simulink model "Xe_Model_Redo_June_26"  (R2018a)
settings: Solver=VariableStepAuto  StartTime=0.0  StopTime=5E5+96*60*60  RelTol=1e-3
values from neighbouring files (symbols this model uses):
  A_pipe = pi*r_pipe^2    (= 0.0126676869774)    [Startup_Script.m]
  alpha_FS = 0.517E-16    (= 5.17e-17)    [Startup_Script.m]
  alpha_G_R1 = 0.334E-17    (= 3.34e-18)    [Startup_Script.m]
  alpha_G_R2 = 0.699E-17    (= 6.99e-18)    [Startup_Script.m]
  alpha_G_R3 = 0.669E-17    (= 6.69e-18)    [Startup_Script.m]
  alpha_G_R4 = 0.791E-18    (= 7.91e-19)    [Startup_Script.m]
  D_g = 2.37E-9    (= 2.37e-09)    [Startup_Script.m]
  epsilon = 0.1    [Startup_Script.m]
  eta_b = 1E-4    (= 0.0001)    [Startup_Script.m]
  eta_fs = 1.2E-4    (= 0.00012)    [Startup_Script.m]
  f_cv = 0.004    [Startup_Script.m]
  FS_Mu_A = 4340    [Startup_Script.m]
  FS_Mu_K = 0.084    [Startup_Script.m]
  FS_Mu_MSRE = 0.007027    [Startup_Script.m]
  FS_rho_A = 3.628    [Startup_Script.m]
  FS_rho_B = 0.00066    [Startup_Script.m]
  FS_rho_MSRE = 2082    [Startup_Script.m]
  gamma_i = 0.0293524    [Startup_Script.m]
  gamma_te = 0.0322482    [Startup_Script.m]
  gamma_xe = 0.00257324    [Startup_Script.m]
  h_fc = 1.6    [Startup_Script.m]
  H_Xe_a = 5.713e-13    [Startup_Script.m]
  H_Xe_b = -7.937e-10    [Startup_Script.m]
  H_Xe_c = 2.809e-07    [Startup_Script.m]
  HX_r_Tube = ((0.5-0.042)/2)*2.54E-2    (= 0.0058166)    [Startup_Script.m]
  HX_XS = HX_N_Tubes*(pi*HX_r_Tube^2)    (= 0.0168999490356)    [Startup_Script.m]
  k_b = 1.3806E-23    (= 1.3806e-23)    [Startup_Script.m]
  lambda_i = 2.9306070546251702E-5    (= 2.93060705463e-05)    [Startup_Script.m]
  lambda_te = 0.036481430555786593    (= 0.0364814305558)    [Startup_Script.m]
  lambda_xe = 2.0924e-05    [Startup_Script.m]
  N_FC_R1 = 12    [Startup_Script.m]
  N_FC_R2 = 940    [Startup_Script.m]
  N_FC_R3 = 108    [Startup_Script.m]
  N_FC_R4 = 78    [Startup_Script.m]
  P_pump = 35420    [Startup_Script.m]
  phi0 = 3.98E+17    (= 3.98e+17)    [Startup_Script.m]
  phi_G_R_1 = mean(interp1(phi_G_R,phi_G_phi, linspace(0,r_g_r1)))    [Startup_Script.m]
  phi_G_R_2 = mean(interp1(phi_G_R,phi_G_phi, linspace(r_g_r1,r_g_r2)))    [Startup_Script.m]
  phi_G_R_3 = mean(interp1(phi_G_R,phi_G_phi, linspace(r_g_r2,r_g_r3)))    [Startup_Script.m]
  phi_G_R_4 = mean(interp1(phi_G_R,phi_G_phi, linspace(r_g_r3,r_g_r4)))    [Startup_Script.m]
  Q_strpr = 0.003155    [Startup_Script.m]
  Q_tot = 0.07571    [Startup_Script.m]
  r_b = 0.000254    [Startup_Script.m]
  r_fc = 0.79e-2    (= 0.0079)    [Startup_Script.m]
  r_pipe = (5E-2*2.54)/2    (= 0.0635)    [Startup_Script.m]
  r_xe = 2.16E-10    (= 2.16e-10)    [Startup_Script.m]
  Re_CA = 25800    [Startup_Script.m]
  Re_LH = 1E4    (= 10000)    [Startup_Script.m]
  Re_UH = 1E4    (= 10000)    [Startup_Script.m]
  sig_a_xe = 1.18E-22    (= 1.18e-22)    [Startup_Script.m]
  Sig_f = 0.15    [Startup_Script.m]
  T_CA_0 = T_INLET    (= 907.594444444)    [Startup_Script.m]
  T_FP_0 = T_OUTLET    (= 935.372222222)    [Startup_Script.m]
  T_FS_R_1_0 = mean(interp1(R_fs_m,T_fs_K, linspace(0,r_g_r1)))    [Startup_Script.m]
  T_FS_R_2_0 = mean(interp1(R_fs_m,T_fs_K, linspace(r_g_r1,r_g_r2)))    [Startup_Script.m]
  T_FS_R_3_0 = mean(interp1(R_fs_m,T_fs_K, linspace(r_g_r2,r_g_r3)))    [Startup_Script.m]
  T_FS_R_4_0 = mean(interp1(R_fs_m,T_fs_K, linspace(r_g_r3,r_g_r4)))    [Startup_Script.m]
  T_G_R_1_0 = mean(interp1(R_gr_m,T_gr_K, linspace(0,r_g_r1)))    [Startup_Script.m]
  T_HX_0 = 0.5*(T_OUTLET + T_INLET)    (= 921.483333333)    [Startup_Script.m]
  T_LH_0 = T_INLET    (= 907.594444444)    [Startup_Script.m]
  T_Mes = 928.15    [Startup_Script.m]
  T_P100_0 = T_OUTLET    (= 935.372222222)    [Startup_Script.m]
  T_P101_0 = T_OUTLET    (= 935.372222222)    [Startup_Script.m]
  T_P102_0 = T_INLET    (= 907.594444444)    [Startup_Script.m]
  T_Salt_0 = 900    [Startup_Script.m]
  T_UH_0 = T_OUTLET    (= 935.372222222)    [Startup_Script.m]
  U_FC_R1 = 0.607    [Startup_Script.m]
  U_FC_R2 = 0.183    [Startup_Script.m]
  U_FC_R3 = 0.454    [Startup_Script.m]
  U_FC_R4 = 0.250    (= 0.25)    [Startup_Script.m]
  V_CA_0 = 9.7*cubed_foot_to_cubed_meter    (= 0.274673445)    [Startup_Script.m]
  V_FP_0 = (0.9+3.2)*cubed_foot_to_cubed_meter    (= 0.116099085)    [Startup_Script.m]
  V_HX_0 = 6.1*cubed_foot_to_cubed_meter    (= 0.172732785)    [Startup_Script.m]
  V_LH_0 = 10.0*cubed_foot_to_cubed_meter    (= 0.2831685)    [Startup_Script.m]
  V_P100_0 = 2.1*cubed_foot_to_cubed_meter    (= 0.059465385)    [Startup_Script.m]
  V_P101_0 = 0.8*cubed_foot_to_cubed_meter    (= 0.02265348)    [Startup_Script.m]
  V_P102_0 = 2.2*cubed_foot_to_cubed_meter    (= 0.06229707)    [Startup_Script.m]
  V_R1_0 = V_Core_FS_0 *N_FC_R1/N_FC_tot    (= 0.00753107712766)    [Startup_Script.m]
  V_R2_0 = V_Core_FS_0 *N_FC_R2/N_FC_tot    (= 0.589934375)    [Startup_Script.m]
  V_R3_0 = V_Core_FS_0 *N_FC_R3/N_FC_tot    (= 0.0677796941489)    [Startup_Script.m]
  V_R4_0 = V_Core_FS_0 *N_FC_R4/N_FC_tot    (= 0.0489520013298)    [Startup_Script.m]
  V_UH_0 = 10.5*cubed_foot_to_cubed_meter    (= 0.297326925)    [Startup_Script.m]
undefined symbols (not defined in the file or in its folder): magnitude, V_CA, V_HX, V_P2, V_P3, V_R1, V_R2, V_R3, V_R4, V_UH
libraries: simulink x4, dspindex x4, dspstat3 x4, SignalEditorBlockLib x2
(part 2 of 11)

== system Xe_Model_Redo_June_26/Graphite /Graphite Region 3 ==
  N_Xe_FS : Inport
  Graphite MTC R1 : Subsystem
  Graphite Stringer : Subsystem
  Product : Product  Inputs=3
  C_Xe_GS_Max : Outport
  C_Xe_GS_Mean : Outport  Port=2
  Nd_Xe_FS->GS : Outport  Port=3
  wires:
  [U_FC_R3] -> Graphite MTC R1/2(U_FC [m/s])
  [phi_G_R_3] -> Graphite Stringer/2(phi)
  [T_G_R_3] -> Graphite MTC R1/1(T_Salt)
  Product/1 -> Nd_Xe_FS->GS/1
  [T_G_R_3] -> Graphite Stringer/1(T)
  N_Xe_FS/1 -> Graphite Stringer/4(N_XE_FS)
  Graphite Stringer/2(C_Xe_GS_Mean) -> C_Xe_GS_Mean/1
  Graphite Stringer/3(J_Xe_FS->GS) -> Product/1
  Graphite Stringer/1(C_Xe_GS_Max) -> C_Xe_GS_Max/1
  [A_1_FC] -> Product/2
  [N_FC_R3] -> Product/3
  Graphite MTC R1/1(k_m_g [m/s]) -> Graphite Stringer/3(k_m_g)

== system Xe_Model_Redo_June_26/Graphite /Graphite Region 4 ==
  N_Xe_FS : Inport
  Graphite MTC R1 : Subsystem
  Graphite Stringer : Subsystem
  Product : Product  Inputs=3
  C_Xe_GS_Max : Outport
  C_Xe_GS_Mean : Outport  Port=2
  Nd_Xe_FS->GS : Outport  Port=3
  wires:
  [U_FC_R4] -> Graphite MTC R1/2(U_FC [m/s])
  [phi_G_R_4] -> Graphite Stringer/2(phi)
  [T_G_R_4] -> Graphite MTC R1/1(T_Salt)
  Product/1 -> Nd_Xe_FS->GS/1
  [T_G_R_4] -> Graphite Stringer/1(T)
  N_Xe_FS/1 -> Graphite Stringer/4(N_XE_FS)
  Graphite Stringer/2(C_Xe_GS_Mean) -> C_Xe_GS_Mean/1
  Graphite Stringer/3(J_Xe_FS->GS) -> Product/1
  Graphite Stringer/1(C_Xe_GS_Max) -> C_Xe_GS_Max/1
  [A_1_FC] -> Product/2
  [N_FC_R4] -> Product/3
  Graphite MTC R1/1(k_m_g [m/s]) -> Graphite Stringer/3(k_m_g)

== system Xe_Model_Redo_June_26/I/I Decay ==
  N_I : Inport
  Product : Product
  Nd_I : Outport
  wires:
  Product/1 -> Nd_I/1
  [lambda_i] -> Product/2
  N_I/1 -> Product/1

== system Xe_Model_Redo_June_26/I/I From Fission ==
  Product : Product  Inputs=4
  Nd_I : Outport
  wires:
  [Sig_f] -> Product/4
  [phi0] -> Product/1
  [gamma_i] -> Product/2
  [V_IC] -> Product/3
  Product/1 -> Nd_I/1

== system Xe_Model_Redo_June_26/Te/Te Decay ==
  n_te : Inport
  Product : Product
  nd_te : Outport
  wires:
  Product/1 -> nd_te/1
  [lambda_te] -> Product/2
  n_te/1 -> Product/1

== system Xe_Model_Redo_June_26/Te/Te From Fission ==
  Product : Product  Inputs=4
  nd_te : Outport
  wires:
  [Sig_f] -> Product/4
  [phi0] -> Product/1
  [gamma_te] -> Product/2
  [V_IC] -> Product/3
  Product/1 -> nd_te/1

== system Xe_Model_Redo_June_26/Xe/Burnout ==
  note: Concentration in all of gas phase
  N_Xe : Inport
  Divide : Product  Inputs=*/
  Product1 : Product  Inputs=4
  Scope1 : Scope
  Scope2 : Scope
  Scope3 : Scope
  Nd_Xe : Outport
  wires:
  [V_FS_liq] -> Divide/2
  Divide/1 -> Product1/1
  [V_IC] -> Scope2/1, Product1/4
  Product1/1 -> Nd_Xe/1
  N_Xe/1 -> Divide/1
  [phi0] -> Scope3/1, Product1/2
  [sig_a_xe] -> Scope1/1, Product1/3

== system Xe_Model_Redo_June_26/Xe/Xe Decay ==
  N_Xe : Inport
  Product : Product
  Nd_Xe : Outport
  wires:
  Product/1 -> Nd_Xe/1
  [lambda_xe] -> Product/2
  N_Xe/1 -> Product/1

== system Xe_Model_Redo_June_26/Xe/Xe From Fission ==
  Product : Product  Inputs=4
  Scope1 : Scope
  Nd_Xe : Outport
  wires:
  [Sig_f] -> Product/4
  [phi0] -> Product/1
  [gamma_xe] -> Product/2
  [V_IC] -> Scope1/1, Product/3
  Product/1 -> Nd_Xe/1

== system Xe_Model_Redo_June_26/Xenon Stripper/Bubble Stripping ==
  Stripper Flowrate [m^3/sec] : Inport
  Bubble Density Bubbles /m^3 : Product  Inputs=*/
  Bubble Flow Rate [bubbles/sec] : Product
  Bubble Removal Rate [Bubbles /sec] : Product
  Bubble Volume Removal Rate [m^3 /sec] : Product
  C_B [atoms/m^3] : Subsystem
  xe removal rate via bubbles [atoms/sec] : Product
  Removal of xenon from bubbles : Outport
  wires:
  [V_CV_Tot] -> Bubble Density Bubbles /m^3/1
  [N_Xe_B] -> C_B [atoms/m^3]/1(N_Xe_B)
  [V_1_B] -> Bubble Density Bubbles /m^3/2
  Bubble Flow Rate [bubbles/sec]/1 -> Bubble Removal Rate [Bubbles /sec]/2
  [eta_b] -> Bubble Removal Rate [Bubbles /sec]/1
  Bubble Removal Rate [Bubbles /sec]/1 -> Bubble Volume Removal Rate [m^3 /sec]/2
  C_B [atoms/m^3]/1(C_Xe_B) -> xe removal rate via bubbles [atoms/sec]/2
  Bubble Density Bubbles /m^3/1 -> Bubble Flow Rate [bubbles/sec]/1
  Stripper Flowrate [m^3/sec]/1 -> Bubble Flow Rate [bubbles/sec]/2
  [V_1_B] -> Bubble Volume Removal Rate [m^3 /sec]/1
  Bubble Volume Removal Rate [m^3 /sec]/1 -> xe removal rate via bubbles [atoms/sec]/1
  xe removal rate via bubbles [atoms/sec]/1 -> Removal of xenon from bubbles/1

== system Xe_Model_Redo_June_26/Xenon Stripper/Fuel Salt Concentration atoms//m^3 ==
  N_FS : Inport
  divide : Product  Inputs=*/
  C_FS : Outport
  wires:
  divide/1 -> C_FS/1
  N_FS/1 -> divide/1
  [V_FS_liq] -> divide/2

== system Xe_Model_Redo_June_26/Xenon Stripper/Fuel Salt Stripping ==
  Stripper Fowrate [m^3/sec] : Inport
  Fuel Salt Concentration [atoms/m^3] : Inport  Port=2
  Product : Product
  atoms/sec : Product
  Fuel Salt Remvoal rate [atoms/sec] : Outport
  wires:
  Product/1 -> Fuel Salt Remvoal rate [atoms/sec]/1
  Fuel Salt Concentration [atoms/m^3]/1 -> atoms/sec/2
  Stripper Fowrate [m^3/sec]/1 -> atoms/sec/1
  atoms/sec/1 -> Product/2
  [eta_fs] -> Product/1

== system Xe_Model_Redo_June_26/Bubbles/Bubble Mass Transfer/Bubble Total KMA ==
  note: Cooling Annulus
  Display7 : Display
      settings: Format=short_e
  HX KMA : Subsystem
  KMA FP : Subsystem
  KMA_CA : Subsystem
  KMA_IC : Subsystem
  KMA_LH : Subsystem
  KMA_UH : Subsystem
  P1 KMA : Subsystem
  P2 KMA : Subsystem
  P3 KMA : Subsystem
  Sum1 : Sum  Inputs=+++++++++
  KMA : Outport
  wires:
  P2 KMA/1(kma) -> Sum1/7
  P1 KMA/1(kma) -> Sum1/5
  KMA_UH/1(kmA) -> Sum1/2
  KMA FP/1(KMA) -> Sum1/6
  KMA_LH/1(kmA) -> Sum1/4
  Sum1/1 -> Display7/1, KMA/1
  KMA_IC/1(kmA) -> Sum1/3
  HX KMA/1(KMA) -> Sum1/8
  KMA_CA/1(KMA) -> Sum1/1
  P3 KMA/1(kma) -> Sum1/9

== system Xe_Model_Redo_June_26/Bubbles/Bubble Mass Transfer/CA ==
  N_Xe FS : Inport
  N_Xe Gas Phase : Inport  Port=2
  T Node : Inport  Port=3
  V_Gas_Node : Inport  Port=4
  Fuel Salt Concentration1 : Subsystem
  "HRT*C_B " : Subsystem
  KMA_CA : Subsystem
  Multiply : Product
  Scope : Scope
  Scope1 : Scope
  Scope2 : Scope
  Subtract1 : Sum  Inputs=+-
  Nd_Xe : Outport
  wires:
  N_Xe FS/1 -> Fuel Salt Concentration1/1(N_FS)
  Multiply/1 -> Nd_Xe/1
  Subtract1/1 -> Scope2/1, Multiply/1
  Fuel Salt Concentration1/1(C_Xe Liq FS) -> Scope/1, Subtract1/1
  V_Gas_Node/1 -> KMA_CA/2(V Gas Node)
  "HRT*C_B "/1(HRT*(C_Xe in Gas Phase)) -> Scope1/1, Subtract1/2
  T Node/1 -> "HRT*C_B "/2(T Node), KMA_CA/1(T FS Node)
  N_Xe Gas Phase/1 -> "HRT*C_B "/1(N_Xe Gas Phase)
  KMA_CA/1(KMA) -> Multiply/2

== system Xe_Model_Redo_June_26/Bubbles/Bubble Mass Transfer/FP ==
  N_Xe FS : Inport
  N_Xe Gas Phase : Inport  Port=2
  T Node : Inport  Port=3
  V_Gas_Node : Inport  Port=4
  Fuel Salt Concentration1 : Subsystem
  "HRT*C_B " : Subsystem
  KMA_FP : Subsystem
  Multiply : Product
  Subtract1 : Sum  Inputs=+-
  Nd_Xe : Outport
  wires:
  N_Xe FS/1 -> Fuel Salt Concentration1/1(N_FS)
  Multiply/1 -> Nd_Xe/1
  Subtract1/1 -> Multiply/1
  Fuel Salt Concentration1/1(C_Xe Liq FS) -> Subtract1/1
  V_Gas_Node/1 -> KMA_FP/2(V Gas Node)
  "HRT*C_B "/1(HRT*(C_Xe in Gas Phase)) -> Subtract1/2
  T Node/1 -> "HRT*C_B "/2(T Node), KMA_FP/1(T FS Node)
  N_Xe Gas Phase/1 -> "HRT*C_B "/1(N_Xe Gas Phase)
  KMA_FP/1(KMA) -> Multiply/2

== system Xe_Model_Redo_June_26/Bubbles/Bubble Mass Transfer/G_R1 ==
  N_Xe FS : Inport
  N_Xe Gas Phase : Inport  Port=2
  T Node : Inport  Port=3
  V_Gas_Node : Inport  Port=4
  Fuel Salt Concentration1 : Subsystem
  "HRT*C_B " : Subsystem
  KMA_G_R1 : Subsystem
  Multiply : Product
  Subtract1 : Sum  Inputs=+-
  Nd_Xe : Outport
  wires:
  N_Xe FS/1 -> Fuel Salt Concentration1/1(N_FS)
  Multiply/1 -> Nd_Xe/1
  Subtract1/1 -> Multiply/1
  Fuel Salt Concentration1/1(C_Xe Liq FS) -> Subtract1/1
  V_Gas_Node/1 -> KMA_G_R1/2(V Gas Node)
  "HRT*C_B "/1(HRT*(C_Xe in Gas Phase)) -> Subtract1/2
  T Node/1 -> KMA_G_R1/1(T FS Node), "HRT*C_B "/2(T Node)
  N_Xe Gas Phase/1 -> "HRT*C_B "/1(N_Xe Gas Phase)
  KMA_G_R1/1(KMA) -> Multiply/2

== system Xe_Model_Redo_June_26/Bubbles/Bubble Mass Transfer/G_R2 ==
  N_Xe FS : Inport
  N_Xe Gas Phase : Inport  Port=2
  T Node : Inport  Port=3
  V_Gas_Node : Inport  Port=4
  Fuel Salt Concentration1 : Subsystem
  "HRT*C_B " : Subsystem
  KMA_G_R1 : Subsystem
  Multiply : Product
  Subtract1 : Sum  Inputs=+-
  Nd_Xe : Outport
  wires:
  N_Xe FS/1 -> Fuel Salt Concentration1/1(N_FS)
  Multiply/1 -> Nd_Xe/1
  Subtract1/1 -> Multiply/1
  Fuel Salt Concentration1/1(C_Xe Liq FS) -> Subtract1/1
  V_Gas_Node/1 -> KMA_G_R1/2(V Gas Node)
  "HRT*C_B "/1(HRT*(C_Xe in Gas Phase)) -> Subtract1/2
  T Node/1 -> KMA_G_R1/1(T FS Node), "HRT*C_B "/2(T Node)
  N_Xe Gas Phase/1 -> "HRT*C_B "/1(N_Xe Gas Phase)
  KMA_G_R1/1(KMA) -> Multiply/2

== system Xe_Model_Redo_June_26/Bubbles/Bubble Mass Transfer/G_R3 ==
  N_Xe FS : Inport
  N_Xe Gas Phase : Inport  Port=2
  T Node : Inport  Port=3
  V_Gas_Node : Inport  Port=4
  Fuel Salt Concentration1 : Subsystem
  "HRT*C_B " : Subsystem
  KMA_G_R1 : Subsystem
  Multiply : Product
  Subtract1 : Sum  Inputs=+-
  Nd_Xe : Outport
  wires:
  N_Xe FS/1 -> Fuel Salt Concentration1/1(N_FS)
  Multiply/1 -> Nd_Xe/1
  Subtract1/1 -> Multiply/1
  Fuel Salt Concentration1/1(C_Xe Liq FS) -> Subtract1/1
  V_Gas_Node/1 -> KMA_G_R1/2(V Gas Node)
  "HRT*C_B "/1(HRT*(C_Xe in Gas Phase)) -> Subtract1/2
  T Node/1 -> KMA_G_R1/1(T FS Node), "HRT*C_B "/2(T Node)
  N_Xe Gas Phase/1 -> "HRT*C_B "/1(N_Xe Gas Phase)
  KMA_G_R1/1(KMA) -> Multiply/2

== system Xe_Model_Redo_June_26/Bubbles/Bubble Mass Transfer/G_R4 ==
  N_Xe FS : Inport
  N_Xe Gas Phase : Inport  Port=2
  T Node : Inport  Port=3
  V_Gas_Node : Inport  Port=4
  Fuel Salt Concentration1 : Subsystem
  "HRT*C_B " : Subsystem
  KMA_G_R1 : Subsystem
  Multiply : Product
  Subtract1 : Sum  Inputs=+-
  Nd_Xe : Outport
  wires:
  N_Xe FS/1 -> Fuel Salt Concentration1/1(N_FS)
  Multiply/1 -> Nd_Xe/1
  Subtract1/1 -> Multiply/1
  Fuel Salt Concentration1/1(C_Xe Liq FS) -> Subtract1/1
  V_Gas_Node/1 -> KMA_G_R1/2(V Gas Node)
  "HRT*C_B "/1(HRT*(C_Xe in Gas Phase)) -> Subtract1/2
  T Node/1 -> KMA_G_R1/1(T FS Node), "HRT*C_B "/2(T Node)
  N_Xe Gas Phase/1 -> "HRT*C_B "/1(N_Xe Gas Phase)
  KMA_G_R1/1(KMA) -> Multiply/2

== system Xe_Model_Redo_June_26/Bubbles/Bubble Mass Transfer/HX ==
  N_Xe FS : Inport
  N_Xe Gas Phase : Inport  Port=2
  T Node : Inport  Port=3
  V_Gas_Node : Inport  Port=4
  Fuel Salt Concentration1 : Subsystem
  "HRT*C_B " : Subsystem
  KMA_HX : Subsystem
  Multiply : Product
  Subtract1 : Sum  Inputs=+-
  Nd_Xe : Outport
  wires:
  N_Xe FS/1 -> Fuel Salt Concentration1/1(N_FS)
  Multiply/1 -> Nd_Xe/1
  Subtract1/1 -> Multiply/1
  Fuel Salt Concentration1/1(C_Xe Liq FS) -> Subtract1/1
  V_Gas_Node/1 -> KMA_HX/2(V Gas Node)
  "HRT*C_B "/1(HRT*(C_Xe in Gas Phase)) -> Subtract1/2
  T Node/1 -> KMA_HX/1(T FS Node), "HRT*C_B "/2(T Node)
  N_Xe Gas Phase/1 -> "HRT*C_B "/1(N_Xe Gas Phase)
  KMA_HX/1(KMA) -> Multiply/2

== system Xe_Model_Redo_June_26/Bubbles/Bubble Mass Transfer/LH ==
  N_Xe FS : Inport
  N_Xe Gas Phase : Inport  Port=2
  T Node : Inport  Port=3
  V_Gas_Node : Inport  Port=4
  Fuel Salt Concentration1 : Subsystem
  "HRT*C_B " : Subsystem
  KMA_LH : Subsystem
  Multiply : Product
  Subtract1 : Sum  Inputs=+-
  Nd_Xe : Outport
  wires:
  N_Xe FS/1 -> Fuel Salt Concentration1/1(N_FS)
  Multiply/1 -> Nd_Xe/1
  Subtract1/1 -> Multiply/1
  Fuel Salt Concentration1/1(C_Xe Liq FS) -> Subtract1/1
  V_Gas_Node/1 -> KMA_LH/2(V Gas Node)
  "HRT*C_B "/1(HRT*(C_Xe in Gas Phase)) -> Subtract1/2
  T Node/1 -> "HRT*C_B "/2(T Node), KMA_LH/1(T FS Node)
  N_Xe Gas Phase/1 -> "HRT*C_B "/1(N_Xe Gas Phase)
  KMA_LH/1(KMA) -> Multiply/2

== system Xe_Model_Redo_June_26/Bubbles/Bubble Mass Transfer/P100 ==
  N_Xe FS : Inport
  N_Xe Gas Phase : Inport  Port=2
  T Node : Inport  Port=3
  V_Gas_Node : Inport  Port=4
  Fuel Salt Concentration1 : Subsystem
  "HRT*C_B " : Subsystem
  KMA_P100 : Subsystem
  Multiply : Product
  Subtract1 : Sum  Inputs=+-
  Nd_Xe : Outport
  wires:
  N_Xe FS/1 -> Fuel Salt Concentration1/1(N_FS)
  Multiply/1 -> Nd_Xe/1
  Subtract1/1 -> Multiply/1
  Fuel Salt Concentration1/1(C_Xe Liq FS) -> Subtract1/1
  V_Gas_Node/1 -> KMA_P100/2(V Gas Node)
  "HRT*C_B "/1(HRT*(C_Xe in Gas Phase)) -> Subtract1/2
  T Node/1 -> KMA_P100/1(T FS Node), "HRT*C_B "/2(T Node)
  N_Xe Gas Phase/1 -> "HRT*C_B "/1(N_Xe Gas Phase)
  KMA_P100/1(KMA) -> Multiply/2

== system Xe_Model_Redo_June_26/Bubbles/Bubble Mass Transfer/P101 ==
  N_Xe FS : Inport
  N_Xe Gas Phase : Inport  Port=2
  T Node : Inport  Port=3
  V_Gas_Node : Inport  Port=4
  Fuel Salt Concentration1 : Subsystem
  "HRT*C_B " : Subsystem
  KMA_P101 : Subsystem
  Multiply : Product
  Subtract1 : Sum  Inputs=+-
  Nd_Xe : Outport
  wires:
  N_Xe FS/1 -> Fuel Salt Concentration1/1(N_FS)
  Multiply/1 -> Nd_Xe/1
  Subtract1/1 -> Multiply/1
  Fuel Salt Concentration1/1(C_Xe Liq FS) -> Subtract1/1
  V_Gas_Node/1 -> KMA_P101/2(V Gas Node)
  "HRT*C_B "/1(HRT*(C_Xe in Gas Phase)) -> Subtract1/2
  T Node/1 -> KMA_P101/1(T FS Node), "HRT*C_B "/2(T Node)
  N_Xe Gas Phase/1 -> "HRT*C_B "/1(N_Xe Gas Phase)
  KMA_P101/1(KMA) -> Multiply/2

== system Xe_Model_Redo_June_26/Bubbles/Bubble Mass Transfer/P102 ==
  N_Xe FS : Inport
  N_Xe Gas Phase : Inport  Port=2
  T Node : Inport  Port=3
  V_Gas_Node : Inport  Port=4
  Fuel Salt Concentration1 : Subsystem
  "HRT*C_B " : Subsystem
  KMA_P102 : Subsystem
  Multiply : Product
  Subtract1 : Sum  Inputs=+-
  Nd_Xe : Outport
  wires:
  N_Xe FS/1 -> Fuel Salt Concentration1/1(N_FS)
  Multiply/1 -> Nd_Xe/1
  Subtract1/1 -> Multiply/1
  Fuel Salt Concentration1/1(C_Xe Liq FS) -> Subtract1/1
  V_Gas_Node/1 -> KMA_P102/2(V Gas Node)
  "HRT*C_B "/1(HRT*(C_Xe in Gas Phase)) -> Subtract1/2
  T Node/1 -> KMA_P102/1(T FS Node), "HRT*C_B "/2(T Node)
  N_Xe Gas Phase/1 -> "HRT*C_B "/1(N_Xe Gas Phase)
  KMA_P102/1(KMA) -> Multiply/2

== system Xe_Model_Redo_June_26/Bubbles/Bubble Mass Transfer/UH ==
  N_Xe FS : Inport
  N_Xe Gas Phase : Inport  Port=2
  T Node : Inport  Port=3
  V_Gas_Node : Inport  Port=4
  Fuel Salt Concentration1 : Subsystem
  "HRT*C_B " : Subsystem
  KMA_UH : Subsystem
  Multiply : Product
  Subtract1 : Sum  Inputs=+-
  Nd_Xe : Outport
  wires:
  N_Xe FS/1 -> Fuel Salt Concentration1/1(N_FS)
  Multiply/1 -> Nd_Xe/1
  Subtract1/1 -> Multiply/1
  Fuel Salt Concentration1/1(C_Xe Liq FS) -> Subtract1/1
  V_Gas_Node/1 -> KMA_UH/2(V Gas Node)
  "HRT*C_B "/1(HRT*(C_Xe in Gas Phase)) -> Subtract1/2
  T Node/1 -> "HRT*C_B "/2(T Node), KMA_UH/1(T FS Node)
  N_Xe Gas Phase/1 -> "HRT*C_B "/1(N_Xe Gas Phase)
  KMA_UH/1(KMA) -> Multiply/2

== system Xe_Model_Redo_June_26/CONSTANTS/V CA/Current Density ==
  T_Salt [k] : Inport
  Cantor F1 Density : Subsystem
  Cantor F1 Density1 : Subsystem
  Constant3 : Constant  Value=T_Mes
  Constant4 : Constant  Value=FS_rho_MSRE
  Divide1 : Product  Inputs=*/
  Product1 : Product
  rho_FS [kg/m^3] : Outport
  wires:
  Divide1/1 -> Product1/2
  Cantor F1 Density1/1(rho [kg/m^3]) -> Divide1/2
  Constant4/1 -> Product1/1
  Cantor F1 Density/1(rho [kg/m^3]) -> Divide1/1
  Product1/1 -> rho_FS [kg/m^3]/1
  Constant3/1 -> Cantor F1 Density1/1(T_Salt [k])
  T_Salt [k]/1 -> Cantor F1 Density/1(T_Salt [k])

== system Xe_Model_Redo_June_26/CONSTANTS/V CA/Gain Gain ==
  Vol. Gas 0 : Inport
  T : Inport  Port=2
  "T_0 " : Inport  Port=3
  Divide : Product  Inputs=*/
  Multiply : Product
  V Gas : Outport
  wires:
  "T_0 "/1 -> Divide/2
  T/1 -> Divide/1
  Multiply/1 -> V Gas/1
  Divide/1 -> Multiply/2
  Vol. Gas 0/1 -> Multiply/1

== system Xe_Model_Redo_June_26/CONSTANTS/V CA/Reference Density ==
  T_Salt [k] : Inport
  Cantor F1 Density : Subsystem
  Cantor F1 Density1 : Subsystem
  Constant3 : Constant  Value=T_Mes
  Constant4 : Constant  Value=FS_rho_MSRE
  Divide1 : Product  Inputs=*/
  Product1 : Product
  rho_FS [kg/m^3] : Outport
  wires:
  Divide1/1 -> Product1/2
  Cantor F1 Density1/1(rho [kg/m^3]) -> Divide1/2
  Constant4/1 -> Product1/1
  Cantor F1 Density/1(rho [kg/m^3]) -> Divide1/1
  Product1/1 -> rho_FS [kg/m^3]/1
  Constant3/1 -> Cantor F1 Density1/1(T_Salt [k])
  T_Salt [k]/1 -> Cantor F1 Density/1(T_Salt [k])

== system Xe_Model_Redo_June_26/CONSTANTS/V FP/Current Density ==
  T_Salt [k] : Inport
  Cantor F1 Density : Subsystem
  Cantor F1 Density1 : Subsystem
  Constant3 : Constant  Value=T_Mes
  Constant4 : Constant  Value=FS_rho_MSRE
  Divide1 : Product  Inputs=*/
  Product1 : Product
  rho_FS [kg/m^3] : Outport
  wires:
  Divide1/1 -> Product1/2
  Cantor F1 Density1/1(rho [kg/m^3]) -> Divide1/2
  Constant4/1 -> Product1/1
  Cantor F1 Density/1(rho [kg/m^3]) -> Divide1/1
  Product1/1 -> rho_FS [kg/m^3]/1
  Constant3/1 -> Cantor F1 Density1/1(T_Salt [k])
  T_Salt [k]/1 -> Cantor F1 Density/1(T_Salt [k])

== system Xe_Model_Redo_June_26/CONSTANTS/V FP/Gain Gain ==
  Vol. Gas 0 : Inport
  T : Inport  Port=2
  "T_0 " : Inport  Port=3
  Divide : Product  Inputs=*/
  Multiply : Product
  V Gas : Outport
  wires:
  "T_0 "/1 -> Divide/2
  T/1 -> Divide/1
  Multiply/1 -> V Gas/1
  Divide/1 -> Multiply/2
  Vol. Gas 0/1 -> Multiply/1

== system Xe_Model_Redo_June_26/CONSTANTS/V FP/Reference Density ==
  T_Salt [k] : Inport
  Cantor F1 Density : Subsystem
  Cantor F1 Density1 : Subsystem
  Constant3 : Constant  Value=T_Mes
  Constant4 : Constant  Value=FS_rho_MSRE
  Divide1 : Product  Inputs=*/
  Product1 : Product
  rho_FS [kg/m^3] : Outport
  wires:
  Divide1/1 -> Product1/2
  Cantor F1 Density1/1(rho [kg/m^3]) -> Divide1/2
  Constant4/1 -> Product1/1
  Cantor F1 Density/1(rho [kg/m^3]) -> Divide1/1
  Product1/1 -> rho_FS [kg/m^3]/1
  Constant3/1 -> Cantor F1 Density1/1(T_Salt [k])
  T_Salt [k]/1 -> Cantor F1 Density/1(T_Salt [k])

== system Xe_Model_Redo_June_26/CONSTANTS/V FP1/Current Density ==
  T_Salt [k] : Inport
  Cantor F1 Density : Subsystem
  Cantor F1 Density1 : Subsystem
  Constant3 : Constant  Value=T_Mes
  Constant4 : Constant  Value=FS_rho_MSRE
  Divide1 : Product  Inputs=*/
  Product1 : Product
  rho_FS [kg/m^3] : Outport
  wires:
  Divide1/1 -> Product1/2
  Cantor F1 Density1/1(rho [kg/m^3]) -> Divide1/2
  Constant4/1 -> Product1/1
  Cantor F1 Density/1(rho [kg/m^3]) -> Divide1/1
  Product1/1 -> rho_FS [kg/m^3]/1
  Constant3/1 -> Cantor F1 Density1/1(T_Salt [k])
  T_Salt [k]/1 -> Cantor F1 Density/1(T_Salt [k])

== system Xe_Model_Redo_June_26/CONSTANTS/V FP1/Gain Gain ==
  Vol. Gas 0 : Inport
  T : Inport  Port=2
  "T_0 " : Inport  Port=3
  Divide : Product  Inputs=*/
  Multiply : Product
  V Gas : Outport
  wires:
  "T_0 "/1 -> Divide/2
  T/1 -> Divide/1
  Multiply/1 -> V Gas/1
  Divide/1 -> Multiply/2
  Vol. Gas 0/1 -> Multiply/1

== system Xe_Model_Redo_June_26/CONSTANTS/V FP1/Reference Density ==
  T_Salt [k] : Inport
  Cantor F1 Density : Subsystem
  Cantor F1 Density1 : Subsystem
  Constant3 : Constant  Value=T_Mes
  Constant4 : Constant  Value=FS_rho_MSRE
  Divide1 : Product  Inputs=*/
  Product1 : Product
  rho_FS [kg/m^3] : Outport
  wires:
  Divide1/1 -> Product1/2
  Cantor F1 Density1/1(rho [kg/m^3]) -> Divide1/2
  Constant4/1 -> Product1/1
  Cantor F1 Density/1(rho [kg/m^3]) -> Divide1/1
  Product1/1 -> rho_FS [kg/m^3]/1
  Constant3/1 -> Cantor F1 Density1/1(T_Salt [k])
  T_Salt [k]/1 -> Cantor F1 Density/1(T_Salt [k])

== system Xe_Model_Redo_June_26/CONSTANTS/V HX/Current Density ==
  T_Salt [k] : Inport
  Cantor F1 Density : Subsystem
  Cantor F1 Density1 : Subsystem
  Constant3 : Constant  Value=T_Mes
  Constant4 : Constant  Value=FS_rho_MSRE
  Divide1 : Product  Inputs=*/
  Product1 : Product
  rho_FS [kg/m^3] : Outport
  wires:
  Divide1/1 -> Product1/2
  Cantor F1 Density1/1(rho [kg/m^3]) -> Divide1/2
  Constant4/1 -> Product1/1
  Cantor F1 Density/1(rho [kg/m^3]) -> Divide1/1
  Product1/1 -> rho_FS [kg/m^3]/1
  Constant3/1 -> Cantor F1 Density1/1(T_Salt [k])
  T_Salt [k]/1 -> Cantor F1 Density/1(T_Salt [k])

== system Xe_Model_Redo_June_26/CONSTANTS/V HX/Gain Gain ==
  Vol. Gas 0 : Inport
  T : Inport  Port=2
  "T_0 " : Inport  Port=3
  Divide : Product  Inputs=*/
  Multiply : Product
  V Gas : Outport
  wires:
  "T_0 "/1 -> Divide/2
  T/1 -> Divide/1
  Multiply/1 -> V Gas/1
  Divide/1 -> Multiply/2
  Vol. Gas 0/1 -> Multiply/1

== system Xe_Model_Redo_June_26/CONSTANTS/V HX/Reference Density ==
  T_Salt [k] : Inport
  Cantor F1 Density : Subsystem
  Cantor F1 Density1 : Subsystem
  Constant3 : Constant  Value=T_Mes
  Constant4 : Constant  Value=FS_rho_MSRE
  Divide1 : Product  Inputs=*/
  Product1 : Product
  rho_FS [kg/m^3] : Outport
  wires:
  Divide1/1 -> Product1/2
  Cantor F1 Density1/1(rho [kg/m^3]) -> Divide1/2
  Constant4/1 -> Product1/1
  Cantor F1 Density/1(rho [kg/m^3]) -> Divide1/1
  Product1/1 -> rho_FS [kg/m^3]/1
  Constant3/1 -> Cantor F1 Density1/1(T_Salt [k])
  T_Salt [k]/1 -> Cantor F1 Density/1(T_Salt [k])

== system Xe_Model_Redo_June_26/CONSTANTS/V LH/Current Density ==
  T_Salt [k] : Inport
  Cantor F1 Density : Subsystem
  Cantor F1 Density1 : Subsystem
  Constant3 : Constant  Value=T_Mes
  Constant4 : Constant  Value=FS_rho_MSRE
  Divide1 : Product  Inputs=*/
  Product1 : Product
  rho_FS [kg/m^3] : Outport
  wires:
  Divide1/1 -> Product1/2
  Cantor F1 Density1/1(rho [kg/m^3]) -> Divide1/2
  Constant4/1 -> Product1/1
  Cantor F1 Density/1(rho [kg/m^3]) -> Divide1/1
  Product1/1 -> rho_FS [kg/m^3]/1
  Constant3/1 -> Cantor F1 Density1/1(T_Salt [k])
  T_Salt [k]/1 -> Cantor F1 Density/1(T_Salt [k])

== system Xe_Model_Redo_June_26/CONSTANTS/V LH/Gain Gain ==
  Vol. Gas 0 : Inport
  T : Inport  Port=2
  "T_0 " : Inport  Port=3
  Divide : Product  Inputs=*/
  Multiply : Product
  V Gas : Outport
  wires:
  "T_0 "/1 -> Divide/2
  T/1 -> Divide/1
  Multiply/1 -> V Gas/1
  Divide/1 -> Multiply/2
  Vol. Gas 0/1 -> Multiply/1

== system Xe_Model_Redo_June_26/CONSTANTS/V LH/Reference Density ==
  T_Salt [k] : Inport
  Cantor F1 Density : Subsystem
  Cantor F1 Density1 : Subsystem
  Constant3 : Constant  Value=T_Mes
  Constant4 : Constant  Value=FS_rho_MSRE
  Divide1 : Product  Inputs=*/
  Product1 : Product
  rho_FS [kg/m^3] : Outport
  wires:
  Divide1/1 -> Product1/2
  Cantor F1 Density1/1(rho [kg/m^3]) -> Divide1/2
  Constant4/1 -> Product1/1
  Cantor F1 Density/1(rho [kg/m^3]) -> Divide1/1
  Product1/1 -> rho_FS [kg/m^3]/1
  Constant3/1 -> Cantor F1 Density1/1(T_Salt [k])
  T_Salt [k]/1 -> Cantor F1 Density/1(T_Salt [k])

== system Xe_Model_Redo_June_26/CONSTANTS/V P100/Current Density ==
  T_Salt [k] : Inport
  Cantor F1 Density : Subsystem
  Cantor F1 Density1 : Subsystem
  Constant3 : Constant  Value=T_Mes
  Constant4 : Constant  Value=FS_rho_MSRE
  Divide1 : Product  Inputs=*/
  Product1 : Product
  rho_FS [kg/m^3] : Outport
  wires:
  Divide1/1 -> Product1/2
  Cantor F1 Density1/1(rho [kg/m^3]) -> Divide1/2
  Constant4/1 -> Product1/1
  Cantor F1 Density/1(rho [kg/m^3]) -> Divide1/1
  Product1/1 -> rho_FS [kg/m^3]/1
  Constant3/1 -> Cantor F1 Density1/1(T_Salt [k])
  T_Salt [k]/1 -> Cantor F1 Density/1(T_Salt [k])

== system Xe_Model_Redo_June_26/CONSTANTS/V P100/Gain Gain ==
  Vol. Gas 0 : Inport
  T : Inport  Port=2
  "T_0 " : Inport  Port=3
  Divide : Product  Inputs=*/
  Multiply : Product
  V Gas : Outport
  wires:
  "T_0 "/1 -> Divide/2
  T/1 -> Divide/1
  Multiply/1 -> V Gas/1
  Divide/1 -> Multiply/2
  Vol. Gas 0/1 -> Multiply/1

== system Xe_Model_Redo_June_26/CONSTANTS/V P100/Reference Density ==
  T_Salt [k] : Inport
  Cantor F1 Density : Subsystem
  Cantor F1 Density1 : Subsystem
  Constant3 : Constant  Value=T_Mes
  Constant4 : Constant  Value=FS_rho_MSRE
  Divide1 : Product  Inputs=*/
  Product1 : Product
  rho_FS [kg/m^3] : Outport
  wires:
  Divide1/1 -> Product1/2
  Cantor F1 Density1/1(rho [kg/m^3]) -> Divide1/2
  Constant4/1 -> Product1/1
  Cantor F1 Density/1(rho [kg/m^3]) -> Divide1/1
  Product1/1 -> rho_FS [kg/m^3]/1
  Constant3/1 -> Cantor F1 Density1/1(T_Salt [k])
  T_Salt [k]/1 -> Cantor F1 Density/1(T_Salt [k])

== system Xe_Model_Redo_June_26/CONSTANTS/V P101/Current Density ==
  T_Salt [k] : Inport
  Cantor F1 Density : Subsystem
  Cantor F1 Density1 : Subsystem
  Constant3 : Constant  Value=T_Mes
  Constant4 : Constant  Value=FS_rho_MSRE
  Divide1 : Product  Inputs=*/
  Product1 : Product
  rho_FS [kg/m^3] : Outport
  wires:
  Divide1/1 -> Product1/2
  Cantor F1 Density1/1(rho [kg/m^3]) -> Divide1/2
  Constant4/1 -> Product1/1
  Cantor F1 Density/1(rho [kg/m^3]) -> Divide1/1
  Product1/1 -> rho_FS [kg/m^3]/1
  Constant3/1 -> Cantor F1 Density1/1(T_Salt [k])
  T_Salt [k]/1 -> Cantor F1 Density/1(T_Salt [k])

== system Xe_Model_Redo_June_26/CONSTANTS/V P101/Gain Gain ==
  Vol. Gas 0 : Inport
  T : Inport  Port=2
  "T_0 " : Inport  Port=3
  Divide : Product  Inputs=*/
  Multiply : Product
  V Gas : Outport
  wires:
  "T_0 "/1 -> Divide/2
  T/1 -> Divide/1
  Multiply/1 -> V Gas/1
  Divide/1 -> Multiply/2
  Vol. Gas 0/1 -> Multiply/1

== system Xe_Model_Redo_June_26/CONSTANTS/V P101/Reference Density ==
  T_Salt [k] : Inport
  Cantor F1 Density : Subsystem
  Cantor F1 Density1 : Subsystem
  Constant3 : Constant  Value=T_Mes
  Constant4 : Constant  Value=FS_rho_MSRE
  Divide1 : Product  Inputs=*/
  Product1 : Product
  rho_FS [kg/m^3] : Outport
  wires:
  Divide1/1 -> Product1/2
  Cantor F1 Density1/1(rho [kg/m^3]) -> Divide1/2
  Constant4/1 -> Product1/1
  Cantor F1 Density/1(rho [kg/m^3]) -> Divide1/1
  Product1/1 -> rho_FS [kg/m^3]/1
  Constant3/1 -> Cantor F1 Density1/1(T_Salt [k])
  T_Salt [k]/1 -> Cantor F1 Density/1(T_Salt [k])

== system Xe_Model_Redo_June_26/CONSTANTS/V P102/Current Density ==
  T_Salt [k] : Inport
  Cantor F1 Density : Subsystem
  Cantor F1 Density1 : Subsystem
  Constant3 : Constant  Value=T_Mes
  Constant4 : Constant  Value=FS_rho_MSRE
  Divide1 : Product  Inputs=*/
  Product1 : Product
  rho_FS [kg/m^3] : Outport
  wires:
  Divide1/1 -> Product1/2
  Cantor F1 Density1/1(rho [kg/m^3]) -> Divide1/2
  Constant4/1 -> Product1/1
  Cantor F1 Density/1(rho [kg/m^3]) -> Divide1/1
  Product1/1 -> rho_FS [kg/m^3]/1
  Constant3/1 -> Cantor F1 Density1/1(T_Salt [k])
  T_Salt [k]/1 -> Cantor F1 Density/1(T_Salt [k])

== system Xe_Model_Redo_June_26/CONSTANTS/V P102/Gain Gain ==
  Vol. Gas 0 : Inport
  T : Inport  Port=2
  "T_0 " : Inport  Port=3
  Divide : Product  Inputs=*/
  Multiply : Product
  V Gas : Outport
  wires:
  "T_0 "/1 -> Divide/2
  T/1 -> Divide/1
  Multiply/1 -> V Gas/1
  Divide/1 -> Multiply/2
  Vol. Gas 0/1 -> Multiply/1

== system Xe_Model_Redo_June_26/CONSTANTS/V P102/Reference Density ==
  T_Salt [k] : Inport
  Cantor F1 Density : Subsystem
  Cantor F1 Density1 : Subsystem
  Constant3 : Constant  Value=T_Mes
  Constant4 : Constant  Value=FS_rho_MSRE
  Divide1 : Product  Inputs=*/
  Product1 : Product
  rho_FS [kg/m^3] : Outport
  wires:
  Divide1/1 -> Product1/2
  Cantor F1 Density1/1(rho [kg/m^3]) -> Divide1/2
  Constant4/1 -> Product1/1
  Cantor F1 Density/1(rho [kg/m^3]) -> Divide1/1
  Product1/1 -> rho_FS [kg/m^3]/1
  Constant3/1 -> Cantor F1 Density1/1(T_Salt [k])
  T_Salt [k]/1 -> Cantor F1 Density/1(T_Salt [k])

== system Xe_Model_Redo_June_26/CONSTANTS/V R1/Current Density ==
  T_Salt [k] : Inport
  Cantor F1 Density : Subsystem
  Cantor F1 Density1 : Subsystem
  Constant3 : Constant  Value=T_Mes
  Constant4 : Constant  Value=FS_rho_MSRE
  Divide1 : Product  Inputs=*/
  Product1 : Product
  rho_FS [kg/m^3] : Outport
  wires:
  Divide1/1 -> Product1/2
  Cantor F1 Density1/1(rho [kg/m^3]) -> Divide1/2
  Constant4/1 -> Product1/1
  Cantor F1 Density/1(rho [kg/m^3]) -> Divide1/1
  Product1/1 -> rho_FS [kg/m^3]/1
  Constant3/1 -> Cantor F1 Density1/1(T_Salt [k])
  T_Salt [k]/1 -> Cantor F1 Density/1(T_Salt [k])

== system Xe_Model_Redo_June_26/CONSTANTS/V R1/Gain Gain ==
  Vol. Gas 0 : Inport
  T : Inport  Port=2
  "T_0 " : Inport  Port=3
  Divide : Product  Inputs=*/
  Multiply : Product
  V Gas : Outport
  wires:
  "T_0 "/1 -> Divide/2
  T/1 -> Divide/1
  Multiply/1 -> V Gas/1
  Divide/1 -> Multiply/2
  Vol. Gas 0/1 -> Multiply/1

== system Xe_Model_Redo_June_26/CONSTANTS/V R1/Reference Density ==
  T_Salt [k] : Inport
  Cantor F1 Density : Subsystem
  Cantor F1 Density1 : Subsystem
  Constant3 : Constant  Value=T_Mes
  Constant4 : Constant  Value=FS_rho_MSRE
  Divide1 : Product  Inputs=*/
  Product1 : Product
  rho_FS [kg/m^3] : Outport
  wires:
  Divide1/1 -> Product1/2
  Cantor F1 Density1/1(rho [kg/m^3]) -> Divide1/2
  Constant4/1 -> Product1/1
  Cantor F1 Density/1(rho [kg/m^3]) -> Divide1/1
  Product1/1 -> rho_FS [kg/m^3]/1
  Constant3/1 -> Cantor F1 Density1/1(T_Salt [k])
  T_Salt [k]/1 -> Cantor F1 Density/1(T_Salt [k])

== system Xe_Model_Redo_June_26/CONSTANTS/V R2/Current Density ==
  T_Salt [k] : Inport
  Cantor F1 Density : Subsystem
  Cantor F1 Density1 : Subsystem
  Constant3 : Constant  Value=T_Mes
  Constant4 : Constant  Value=FS_rho_MSRE
  Divide1 : Product  Inputs=*/
  Product1 : Product
  rho_FS [kg/m^3] : Outport
  wires:
  Divide1/1 -> Product1/2
  Cantor F1 Density1/1(rho [kg/m^3]) -> Divide1/2
  Constant4/1 -> Product1/1
  Cantor F1 Density/1(rho [kg/m^3]) -> Divide1/1
  Product1/1 -> rho_FS [kg/m^3]/1
  Constant3/1 -> Cantor F1 Density1/1(T_Salt [k])
  T_Salt [k]/1 -> Cantor F1 Density/1(T_Salt [k])

== system Xe_Model_Redo_June_26/CONSTANTS/V R2/Gain Gain ==
  Vol. Gas 0 : Inport
  T : Inport  Port=2
  "T_0 " : Inport  Port=3
  Divide : Product  Inputs=*/
  Multiply : Product
  V Gas : Outport
  wires:
  "T_0 "/1 -> Divide/2
  T/1 -> Divide/1
  Multiply/1 -> V Gas/1
  Divide/1 -> Multiply/2
  Vol. Gas 0/1 -> Multiply/1

== system Xe_Model_Redo_June_26/CONSTANTS/V R2/Reference Density ==
  T_Salt [k] : Inport
  Cantor F1 Density : Subsystem
  Cantor F1 Density1 : Subsystem
  Constant3 : Constant  Value=T_Mes
  Constant4 : Constant  Value=FS_rho_MSRE
  Divide1 : Product  Inputs=*/
  Product1 : Product
  rho_FS [kg/m^3] : Outport
  wires:
  Divide1/1 -> Product1/2
  Cantor F1 Density1/1(rho [kg/m^3]) -> Divide1/2
  Constant4/1 -> Product1/1
  Cantor F1 Density/1(rho [kg/m^3]) -> Divide1/1
  Product1/1 -> rho_FS [kg/m^3]/1
  Constant3/1 -> Cantor F1 Density1/1(T_Salt [k])
  T_Salt [k]/1 -> Cantor F1 Density/1(T_Salt [k])

== system Xe_Model_Redo_June_26/CONSTANTS/V R3/Current Density ==
  T_Salt [k] : Inport
  Cantor F1 Density : Subsystem
  Cantor F1 Density1 : Subsystem
  Constant3 : Constant  Value=T_Mes
  Constant4 : Constant  Value=FS_rho_MSRE
  Divide1 : Product  Inputs=*/
  Product1 : Product
  rho_FS [kg/m^3] : Outport
  wires:
  Divide1/1 -> Product1/2
  Cantor F1 Density1/1(rho [kg/m^3]) -> Divide1/2
  Constant4/1 -> Product1/1
  Cantor F1 Density/1(rho [kg/m^3]) -> Divide1/1
  Product1/1 -> rho_FS [kg/m^3]/1
  Constant3/1 -> Cantor F1 Density1/1(T_Salt [k])
  T_Salt [k]/1 -> Cantor F1 Density/1(T_Salt [k])

== system Xe_Model_Redo_June_26/CONSTANTS/V R3/Gain Gain ==
  Vol. Gas 0 : Inport
  T : Inport  Port=2
  "T_0 " : Inport  Port=3
  Divide : Product  Inputs=*/
  Multiply : Product
  V Gas : Outport
  wires:
  "T_0 "/1 -> Divide/2
  T/1 -> Divide/1
  Multiply/1 -> V Gas/1
  Divide/1 -> Multiply/2
  Vol. Gas 0/1 -> Multiply/1

== system Xe_Model_Redo_June_26/CONSTANTS/V R3/Reference Density ==
  T_Salt [k] : Inport
  Cantor F1 Density : Subsystem
  Cantor F1 Density1 : Subsystem
  Constant3 : Constant  Value=T_Mes
  Constant4 : Constant  Value=FS_rho_MSRE
  Divide1 : Product  Inputs=*/
  Product1 : Product
  rho_FS [kg/m^3] : Outport
  wires:
  Divide1/1 -> Product1/2
  Cantor F1 Density1/1(rho [kg/m^3]) -> Divide1/2
  Constant4/1 -> Product1/1
  Cantor F1 Density/1(rho [kg/m^3]) -> Divide1/1
  Product1/1 -> rho_FS [kg/m^3]/1
  Constant3/1 -> Cantor F1 Density1/1(T_Salt [k])
  T_Salt [k]/1 -> Cantor F1 Density/1(T_Salt [k])

== system Xe_Model_Redo_June_26/CONSTANTS/V R4/Current Density ==
  T_Salt [k] : Inport
  Cantor F1 Density : Subsystem
  Cantor F1 Density1 : Subsystem
  Constant3 : Constant  Value=T_Mes
  Constant4 : Constant  Value=FS_rho_MSRE
  Divide1 : Product  Inputs=*/
  Product1 : Product
  rho_FS [kg/m^3] : Outport
  wires:
  Divide1/1 -> Product1/2
  Cantor F1 Density1/1(rho [kg/m^3]) -> Divide1/2
  Constant4/1 -> Product1/1
  Cantor F1 Density/1(rho [kg/m^3]) -> Divide1/1
  Product1/1 -> rho_FS [kg/m^3]/1
  Constant3/1 -> Cantor F1 Density1/1(T_Salt [k])
  T_Salt [k]/1 -> Cantor F1 Density/1(T_Salt [k])

== system Xe_Model_Redo_June_26/CONSTANTS/V R4/Gain Gain ==
  Vol. Gas 0 : Inport
  T : Inport  Port=2
  "T_0 " : Inport  Port=3
  Divide : Product  Inputs=*/
  Multiply : Product
  V Gas : Outport
  wires:
  "T_0 "/1 -> Divide/2
  T/1 -> Divide/1
  Multiply/1 -> V Gas/1
  Divide/1 -> Multiply/2
  Vol. Gas 0/1 -> Multiply/1

== system Xe_Model_Redo_June_26/CONSTANTS/V R4/Reference Density ==
  T_Salt [k] : Inport
  Cantor F1 Density : Subsystem
  Cantor F1 Density1 : Subsystem
  Constant3 : Constant  Value=T_Mes
  Constant4 : Constant  Value=FS_rho_MSRE
  Divide1 : Product  Inputs=*/
  Product1 : Product
  rho_FS [kg/m^3] : Outport
  wires:
  Divide1/1 -> Product1/2
  Cantor F1 Density1/1(rho [kg/m^3]) -> Divide1/2
  Constant4/1 -> Product1/1
  Cantor F1 Density/1(rho [kg/m^3]) -> Divide1/1
  Product1/1 -> rho_FS [kg/m^3]/1
  Constant3/1 -> Cantor F1 Density1/1(T_Salt [k])
  T_Salt [k]/1 -> Cantor F1 Density/1(T_Salt [k])

== system Xe_Model_Redo_June_26/CONSTANTS/V UH/Current Density ==
  T_Salt [k] : Inport
  Cantor F1 Density : Subsystem
  Cantor F1 Density1 : Subsystem
  Constant3 : Constant  Value=T_Mes
  Constant4 : Constant  Value=FS_rho_MSRE
  Divide1 : Product  Inputs=*/
  Product1 : Product
  rho_FS [kg/m^3] : Outport
  wires:
  Divide1/1 -> Product1/2
  Cantor F1 Density1/1(rho [kg/m^3]) -> Divide1/2
  Constant4/1 -> Product1/1
  Cantor F1 Density/1(rho [kg/m^3]) -> Divide1/1
  Product1/1 -> rho_FS [kg/m^3]/1
  Constant3/1 -> Cantor F1 Density1/1(T_Salt [k])
  T_Salt [k]/1 -> Cantor F1 Density/1(T_Salt [k])

== system Xe_Model_Redo_June_26/CONSTANTS/V UH/Gain Gain ==
  Vol. Gas 0 : Inport
  T : Inport  Port=2
  "T_0 " : Inport  Port=3
  Divide : Product  Inputs=*/
  Multiply : Product
  V Gas : Outport
  wires:
  "T_0 "/1 -> Divide/2
  T/1 -> Divide/1
  Multiply/1 -> V Gas/1
  Divide/1 -> Multiply/2
  Vol. Gas 0/1 -> Multiply/1

== system Xe_Model_Redo_June_26/CONSTANTS/V UH/Reference Density ==
  T_Salt [k] : Inport
  Cantor F1 Density : Subsystem
  Cantor F1 Density1 : Subsystem
  Constant3 : Constant  Value=T_Mes
  Constant4 : Constant  Value=FS_rho_MSRE
  Divide1 : Product  Inputs=*/
  Product1 : Product
  rho_FS [kg/m^3] : Outport
  wires:
  Divide1/1 -> Product1/2
  Cantor F1 Density1/1(rho [kg/m^3]) -> Divide1/2
  Constant4/1 -> Product1/1
  Cantor F1 Density/1(rho [kg/m^3]) -> Divide1/1
  Product1/1 -> rho_FS [kg/m^3]/1
  Constant3/1 -> Cantor F1 Density1/1(T_Salt [k])
  T_Salt [k]/1 -> Cantor F1 Density/1(T_Salt [k])

== system Xe_Model_Redo_June_26/Graphite /Graphite Region 1/Graphite MTC R1 ==
  note: Diemnsionless Numbers
  note: Thermophysical Properties
  T_Salt : Inport
  U_FC [m/s] : Inport  Port=2
  Constant : Constant  Value=0.023
  Constant1 : Constant  Value=0.8
  Constant2 : Constant  Value=0.4
  Density W Scaling : Subsystem
  Display : Display
  Divide : Product  Inputs=*/
  Gain : Gain  Gain=2
  Mass Diffusion Coeffecient [m^2 /s] : Subsystem
  Math Function : Math  Operator=pow  SaturateOnIntegerOverflow=on
  Math Function1 : Math  Operator=pow  SaturateOnIntegerOverflow=on
  Product : Product
  Reynolds Number : Subsystem
  Schmidt Number : Subsystem
  Sherwood Number : Product  Inputs=3
  Viscosity W Scaling : Subsystem
  k_m_g [m/s] : Outport
  wires:
  [D_FS_Local] -> Divide/1
  Constant2/1 -> Math Function1/2
  [r_fc] -> Gain/1
  Constant/1 -> Sherwood Number/1
  Sherwood Number/1 -> Product/1
  [Sc_FC_Local] -> Math Function1/1
  Divide/1 -> Product/2
  Math Function/1 -> Sherwood Number/2
  Constant1/1 -> Math Function/2
  Product/1 -> k_m_g [m/s]/1
  [Re_FC_Local] -> Math Function/1
  Math Function1/1 -> Sherwood Number/3
  Viscosity W Scaling/1(mu [Pa-s]) -> Mass Diffusion Coeffecient [m^2 /s]/1(Mu), [Mu_FS_Local]
  Density W Scaling/1(rho_FS [kg/m^3]) -> [Rho_FS_Local]
  Mass Diffusion Coeffecient [m^2 /s]/1(D [m^2/s]) -> [D_FS_Local]
  T_Salt/1 -> Mass Diffusion Coeffecient [m^2 /s]/2(T_Salt [k]), Density W Scaling/1(T_Salt [k]), Viscosity W Scaling/1(T_Salt [k])
  Schmidt Number/1(Sc) -> [Sc_FC_Local]
  Reynolds Number/1(Re) -> Display/1, [Re_FC_Local]
  U_FC [m/s]/1 -> Reynolds Number/1(Flow_Velocity [m/s])
  [Rho_FS_Local] -> Reynolds Number/2(rho [kg/m^3])
  [Mu_FS_Local] -> Reynolds Number/3(mu [Pa s])
  [Mu_FS_Local] -> Schmidt Number/1(mu [Pa s])
  [Rho_FS_Local] -> Schmidt Number/2(rho [kg/m^3])
  [D_FS_Local] -> Schmidt Number/3(D [m^2/s])
  Gain/1 -> Divide/2

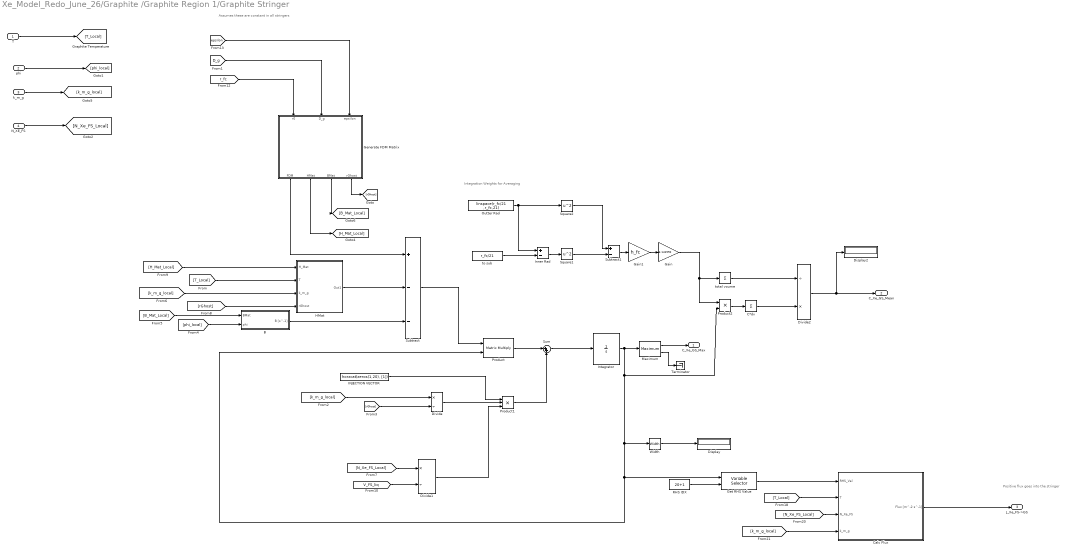
== system Xe_Model_Redo_June_26/Graphite /Graphite Region 1/Graphite Stringer ==
  note: Integration Weights for Averaging
  note: Assumes these are constant in all stringers
  note: Positive flux goes into the stringer
  T : Inport
  phi : Inport  Port=2
  k_m_g : Inport  Port=3
  N_XE_FS : Inport  Port=4
  B : Subsystem
  C*dv : Sum  Inputs=+
  Calc Flux : Subsystem
  Display : Display
  Display2 : Display
  Divide : Product  Inputs=*/
  Divide1 : Product  Inputs=*/
  Divide2 : Product  Inputs=/*
  Gain : Gain  Gain=3.141592
  Gain1 : Gain  Gain=h_fc
  "Generate FDM Matrix " : MATLAB Function  TreatAsAtomicUnit=on
  Get RHS Value : dspindex/Variable Selector  NumInputs=1  rowsOrCols=Rows  IdxMode=Variable  Elements=[1 3]  ZerOneIdxMode=One-based  errmode=Clip Index  FillMode=on  FillValues=0
  HMat : Subsystem
  INJECTION VECTOR : Constant  Value=horzcat(zeros(1,20), [1])
  Inner Rad : Sum  Inputs=+-
  Integrator : Integrator
  Maximum : dspstat3/Maximum  operation=maximum  fcn=Value and Index  indexBase=One  operateOver=Each column  Dimension=1  InputProcessing=Columns as channels (frame based)  reset=None  roiEnable=off  roiType=Rectangles  roiPortion=Entire ROI  roiOutput=Individual statistics for each ROI  roiFlag=off  roundingMode=Floor  overflowMode=off  accumDataTypeStr=Inherit: Same as product output  accumLastDataTypeStr=Inherit: Same as product output
  Outter Rad : Constant  Value=linspace(r_fc/21 ,r_fc,21)
  Product : Product  Multiplication=Matrix(*)
  Product1 : Product  Inputs=3
  Product2 : Product
  RHS IDX : Constant  Value=20+1
  Square1 : Math  Operator=square  SaturateOnIntegerOverflow=on
  Square2 : Math  Operator=square  SaturateOnIntegerOverflow=on
  Subtract : Sum  Inputs=+--
  Subtract1 : Sum  Inputs=+-
  Sum : Sum  Inputs=|++
  Terminator : Terminator
  Width : Width
  to sub : Constant  Value=r_fc/21
  total voume : Sum  Inputs=+
  C_Xe_GS_Max : Outport
  C_Xe_GS_Mean : Outport  Port=2
  J_Xe_FS->GS : Outport  Port=3
  wires:
  Get RHS Value/1 -> Calc Flux/1(RHS_Val)
  Calc Flux/1("Flux [m^-2 s^-1] ") -> J_Xe_FS->GS/1
  HMat/1(Out1) -> Subtract/2
  Maximum/1 -> C_Xe_GS_Max/1
  [rGhost] -> Divide/2
  Divide/1 -> Product1/2
  "Generate FDM Matrix "/1(FDM) -> Subtract/1
  "Generate FDM Matrix "/4(rGhost) -> [rGhost]
  [B_Mat_Local] -> B/1(BMat)
  phi/1 -> [phi_local]
  Subtract/1 -> Product/1
  Divide1/1 -> Product1/3
  Integrator/1 -> Product2/2, Width/1, Product/2, Get RHS Value/1, Maximum/1
  INJECTION VECTOR/1 -> Product1/1
  Product/1 -> Sum/1
  [T_Local] -> HMat/2(T)
  [epsilon] -> "Generate FDM Matrix "/3(epsilon)
  k_m_g/1 -> [k_m_g_local]
  [phi_local] -> B/2(phi)
  [k_m_g_local] -> HMat/3(k_m_g)
  [D_g] -> "Generate FDM Matrix "/2(D_g)
  "Generate FDM Matrix "/3(BMat) -> [B_Mat_Local]
  T/1 -> [T_Local]
  "Generate FDM Matrix "/2(HMat) -> [H_Mat_Local]
  [H_Mat_Local] -> HMat/1(H_Mat)
  [rGhost] -> HMat/4(rGhost)
  [k_m_g_local] -> Divide/1
  [r_fc] -> "Generate FDM Matrix "/1(r0)
  B/1("B [s^-1] ") -> Subtract/3
  Product1/1 -> Sum/2
  Sum/1 -> Integrator/1
  [V_FS_liq] -> Divide1/2
  RHS IDX/1 -> Get RHS Value/2
  [T_Local] -> Calc Flux/2(T)
  N_XE_FS/1 -> [N_Xe_FS_Local]
  [N_Xe_FS_Local] -> Divide1/1
  [k_m_g_local] -> Calc Flux/4(k_m_g)
  [N_Xe_FS_Local] -> Calc Flux/3(N_Xe_FS)
  Width/1 -> Display/1
  Outter Rad/1 -> Inner Rad/1, Square2/1
  Subtract1/1 -> Gain1/1
  Square1/1 -> Subtract1/2
  Square2/1 -> Subtract1/1
  Gain1/1 -> Gain/1
  to sub/1 -> Inner Rad/2
  Inner Rad/1 -> Square1/1
  Gain/1 -> Product2/1, total voume/1
  total voume/1 -> Divide2/1
  Product2/1 -> C*dv/1
  Divide2/1 -> Display2/1, C_Xe_GS_Mean/1
  C*dv/1 -> Divide2/2
  Maximum/2 -> Terminator/1

== system Xe_Model_Redo_June_26/Graphite /Graphite Region 1/Lumped Parameter Graphite Model ==
  PDE : Inport
  In2 : Inport  Port=2
  In3 : Inport  Port=3
  In4 : Inport  Port=4
  Burnout : Subsystem
  Constant : Constant  Value=h_fc
  Constant1 : Constant  Value=3.141592
  Divide : Product  Inputs=*/
  Integrator : Integrator
  Mux : Mux  Inputs=2
  Product1 : Product  Inputs=3
  Square1 : Math  Operator=square  SaturateOnIntegerOverflow=on
  Subsystem : Subsystem
  Sum : Sum  Inputs=+--
  To Workspace : ToWorkspace  VariableName=toSave_PDE  SampleTime=-1
  To Workspace1 : ToWorkspace  VariableName=toSave_LP  SampleTime=-1
  Xe Decay : Subsystem
  Out1 : Outport
  tag scope: V_GS=global
  wires:
  In3/1 -> Subsystem/2(MTC)
  [V_GS] -> Divide/2
  Constant/1 -> Product1/2
  [A_1_FC] -> Subsystem/5(A)
  Divide/1 -> To Workspace1/1, Mux/2  "LP"
  Product1/1 -> [V_GS]
  In2/1 -> Subsystem/1(T)
  Square1/1 -> Product1/1
  PDE/1 -> To Workspace/1, Mux/1
  [r_fc] -> Square1/1
  Subsystem/1(Out1) -> Sum/1
  Burnout/1(Nd_Xe) -> Sum/2
  Integrator/1 -> Divide/1, Xe Decay/1(N_Xe_B), Subsystem/4(N_Xe_G), Burnout/1(N_Xe_G)
  Xe Decay/1(Nd_Xe) -> Sum/3
  [phi_G_R_1] -> Burnout/2(Phi)
  Sum/1 -> Integrator/1
  Constant1/1 -> Product1/3
  In4/1 -> Subsystem/3(V_FS_liq)
  Mux/1 -> Out1/1

== system Xe_Model_Redo_June_26/Graphite /Graphite Region 2/Graphite MTC R1 ==
  note: Diemnsionless Numbers
  note: Thermophysical Properties
  T_Salt : Inport
  U_FC [m/s] : Inport  Port=2
  Constant : Constant  Value=0.023
  Constant1 : Constant  Value=0.8
  Constant2 : Constant  Value=0.4
  Density W Scaling : Subsystem
  Display : Display
  Divide : Product  Inputs=*/
  Gain : Gain  Gain=2
  Mass Diffusion Coeffecient [m^2 /s] : Subsystem
  Math Function : Math  Operator=pow  SaturateOnIntegerOverflow=on
  Math Function1 : Math  Operator=pow  SaturateOnIntegerOverflow=on
  Product : Product
  Reynolds Number : Subsystem
  Schmidt Number : Subsystem
  Sherwood Number : Product  Inputs=3
  Viscosity W Scaling : Subsystem
  k_m_g [m/s] : Outport
  wires:
  [D_FS_Local] -> Divide/1
  Constant2/1 -> Math Function1/2
  [r_fc] -> Gain/1
  Constant/1 -> Sherwood Number/1
  Sherwood Number/1 -> Product/1
  [Sc_FC_Local] -> Math Function1/1
  Divide/1 -> Product/2
  Math Function/1 -> Sherwood Number/2
  Constant1/1 -> Math Function/2
  Product/1 -> k_m_g [m/s]/1
  [Re_FC_Local] -> Math Function/1
  Math Function1/1 -> Sherwood Number/3
  Viscosity W Scaling/1(mu [Pa-s]) -> Mass Diffusion Coeffecient [m^2 /s]/1(Mu), [Mu_FS_Local]
  Density W Scaling/1(rho_FS [kg/m^3]) -> [Rho_FS_Local]
  Mass Diffusion Coeffecient [m^2 /s]/1(D [m^2/s]) -> [D_FS_Local]
  T_Salt/1 -> Mass Diffusion Coeffecient [m^2 /s]/2(T_Salt [k]), Density W Scaling/1(T_Salt [k]), Viscosity W Scaling/1(T_Salt [k])
  Schmidt Number/1(Sc) -> [Sc_FC_Local]
  Reynolds Number/1(Re) -> Display/1, [Re_FC_Local]
  U_FC [m/s]/1 -> Reynolds Number/1(Flow_Velocity [m/s])
  [Rho_FS_Local] -> Reynolds Number/2(rho [kg/m^3])
  [Mu_FS_Local] -> Reynolds Number/3(mu [Pa s])
  [Mu_FS_Local] -> Schmidt Number/1(mu [Pa s])
  [Rho_FS_Local] -> Schmidt Number/2(rho [kg/m^3])
  [D_FS_Local] -> Schmidt Number/3(D [m^2/s])
  Gain/1 -> Divide/2
